simulink model "velo_test"  (Simulink 7.9)
settings: Solver=FixedStepDiscrete  StartTime=0.0  StopTime=10.0  RelTol=1e-3
values from neighbouring files (symbols this model uses):
  ts = 1/50    (= 0.02)    [velo_id_gain.m]    (also in velo_id_tc.m; velo_pi_mbd.m)
libraries: arduino_io_lib x5
settings Model: Creator=hirata  LastModifiedBy=hirata

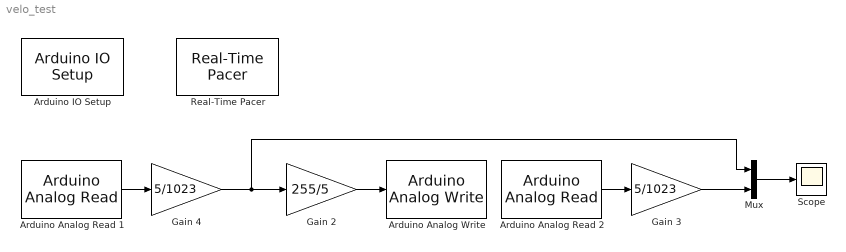
== system velo_test ==
  Arduino Analog Read 1 : arduino_io_lib/Arduino Analog Read  arduinoVar=Temporary arduino variable: Arduino1  arduinoPin=1  T=ts
  Arduino Analog Read 2 : arduino_io_lib/Arduino Analog Read  arduinoVar=Temporary arduino variable: Arduino1  arduinoPin=0  T=ts
  Arduino Analog Write : arduino_io_lib/Arduino Analog Write  arduinoVar=Temporary arduino variable: Arduino1  arduinoPin=3  T=ts
  Arduino IO Setup : arduino_io_lib/Arduino IO Setup  Priority=3  arduinoVar=Temporary arduino variable: Arduino1  workspaceVarName=a  comPort=COM3
  Gain 2 : Gain  Gain=255/5
  Gain 3 : Gain  Gain=5/1023
  Gain 4 : Gain  Gain=5/1023
  Mux : Mux  Inputs=2
  Real-Time Pacer : arduino_io_lib/Real-Time Pacer  simTimePerRealTime=1
  Scope : Scope
      settings: TimeRange=10  YMin=0
  wires:
  Arduino Analog Read 2/1 -> Gain 3/1
  Gain 2/1 -> Arduino Analog Write/1
  Gain 3/1 -> Mux/2
  Mux/1 -> Scope/1
  Arduino Analog Read 1/1 -> Gain 4/1
  Gain 4/1 -> Gain 2/1, Mux/1
